simulink model "Model"  (R2020b)
settings: Solver=VariableStepAuto  StartTime=0.0  StopTime=120  RelTol=1e-3
PreLoadFcn:
  | vars
model workspace: external: MATLAB File C:\Users\hp\MATLAB\Projects\week_2\Project_2\vars.m (data not in the file)
values from neighbouring files (symbols this model uses):
  b = 50    [variables.m]
  m = 1000    [variables.m]
settings Model: DataDictionary=problem_3.sldd  Creator=hp  LastModifiedBy=hp
settings DebuggingCC: ModelReferenceExtraNoncontSigs=none

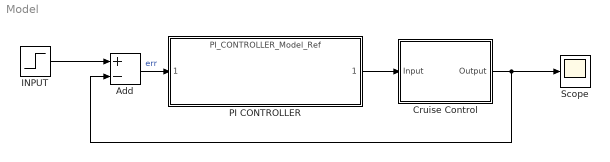
== system Model ==
  Add : Sum  Inputs=+-
  Cruise Control : Subsystem
  INPUT : Step  Time=0  After=u  SampleTime=0
  PI CONTROLLER : ModelReference  ModelNameDialog=PI_CONTROLLER_Model_Ref  UsingDefaultArgumentValue=0,0  SimulationMode=Normal  ModelReferenceVersion=1.20  Ki=0.185  Kp=2.28  SimulationMode=Normal
  Scope : Scope
  wires:
  Cruise Control/1(Output) -> Add/2, Scope/1
  Add/1 -> PI CONTROLLER/1  "err"
  INPUT/1 -> Add/1
  PI CONTROLLER/1 -> Cruise Control/1(Input)

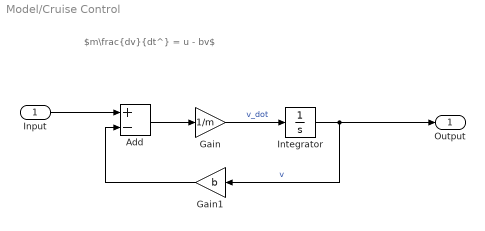
== system Model/Cruise Control ==
  note: $m\frac{dv}{dt^} = u - bv$
  Input : Inport
  Add : Sum  Inputs=+-
  Gain : Gain  Gain=1/m
  Gain1 : Gain  Gain=b
  Integrator : Integrator
  Output : Outport
  wires:
  Integrator/1 -> Output/1, Gain1/1  "v"
  Add/1 -> Gain/1
  Input/1 -> Add/1
  Gain/1 -> Integrator/1  "v_dot"
  Gain1/1 -> Add/2
